simulink model "Observador_discreto"  (R2021a)
settings: Solver=VariableStepAuto  StartTime=0.0  StopTime=10.0  RelTol=1e-3
undefined symbols (not defined in the file): Jeq, Ke_i, Ke_theta, Ke_w, ts
settings Model: Creator=fhlla  LastModifiedBy=fhlla

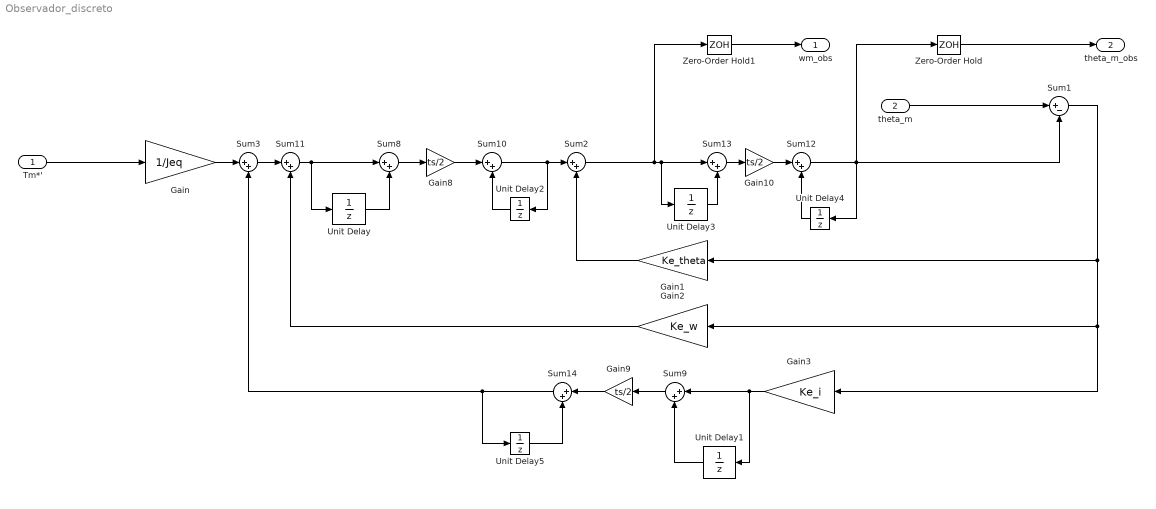
== system Observador_discreto ==
  Tm*' : Inport
  theta_m : Inport  Port=2
  Gain : Gain  Gain=1/Jeq
  Gain1 : Gain  Gain=Ke_theta
  Gain10 : Gain  Gain=ts/2
  Gain2 : Gain  Gain=Ke_w
  Gain3 : Gain  Gain=Ke_i
  Gain8 : Gain  Gain=ts/2
  Gain9 : Gain  Gain=ts/2
  Sum1 : Sum  Inputs=|+-
  Sum{2..3,8..14} (9 alike) : Sum  Inputs=|++
  Unit Delay{,1..5} (6 alike) : UnitDelay  SampleTime=-1  HasFrameUpgradeWarning=on
  Zero-Order Hold : ZeroOrderHold  SampleTime=-1
  Zero-Order Hold1 : ZeroOrderHold  SampleTime=-1
  wm_obs : Outport
  theta_m_obs : Outport  Port=2
  wires:
  Sum12/1 -> Zero-Order Hold/1, Unit Delay4/1, Sum1/2
  Sum8/1 -> Gain8/1
  Unit Delay1/1 -> Sum9/2
  Sum2/1 -> Sum13/1, Unit Delay3/1, Zero-Order Hold1/1
  Sum1/1 -> Gain1/1, Gain3/1, Gain2/1
  Gain9/1 -> Sum14/1
  Sum9/1 -> Gain9/1
  Unit Delay3/1 -> Sum13/2
  Gain1/1 -> Sum2/2
  Sum3/1 -> Sum11/1
  Sum14/1 -> Unit Delay5/1, Sum3/2
  Gain10/1 -> Sum12/1
  Gain2/1 -> Sum11/2
  Gain/1 -> Sum3/1
  Zero-Order Hold1/1 -> wm_obs/1
  Sum10/1 -> Unit Delay2/1, Sum2/1
  Sum11/1 -> Unit Delay/1, Sum8/1
  Tm*'/1 -> Gain/1
  Unit Delay4/1 -> Sum12/2
  Unit Delay2/1 -> Sum10/2
  Zero-Order Hold/1 -> theta_m_obs/1
  Gain8/1 -> Sum10/1
  Gain3/1 -> Unit Delay1/1, Sum9/1
  theta_m/1 -> Sum1/1
  Unit Delay5/1 -> Sum14/2
  Unit Delay/1 -> Sum8/2
  Sum13/1 -> Gain10/1
